simulink model "RadarSimulation"  (R2024a)
settings: Solver=VariableStepAuto  StartTime=0.0  StopTime=10.0  RelTol=1e-3
undefined symbols (not defined in the file or in its folder): physconst, pulseCoefficients
libraries: phasedenvlib x2, phasedtxrxlib x2, phaseddetectlib x1, dspxfrm3 x1
settings Model: Creator=Jayashre  LastModifiedBy=Jayashre

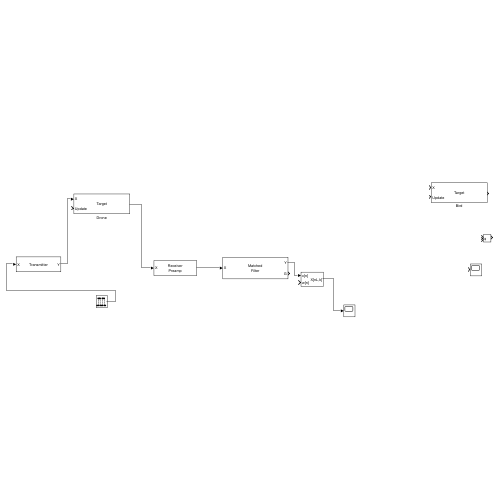
[thumbnail: Simulink's stored preview of the top-level diagram]
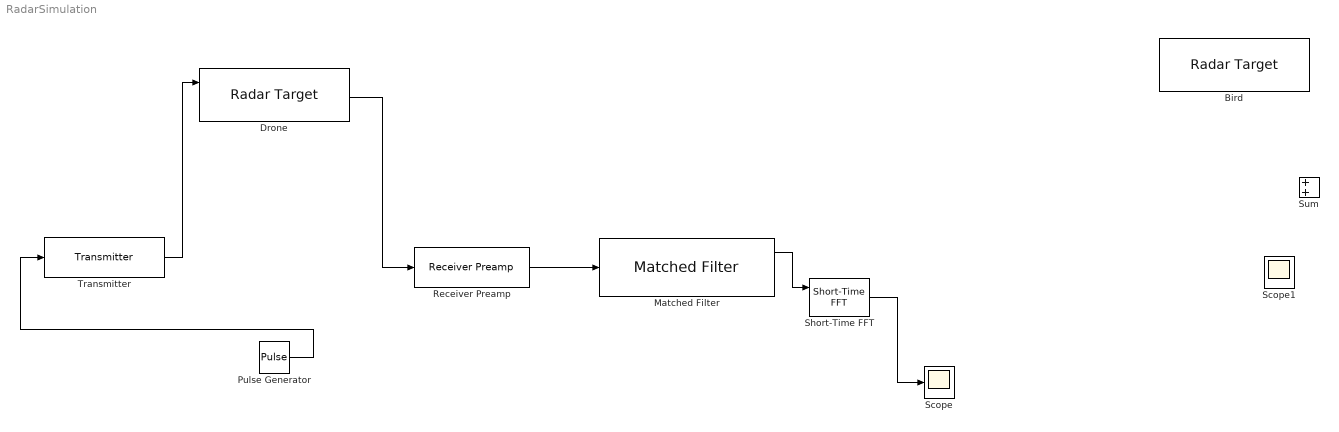
== system RadarSimulation ==
  Bird : phasedenvlib/Radar Target  EnablePolarization=off  Mode=Monostatic  MeanRCSSource=Property  ScatteringMatrixSource=Property  MeanRCS=0.01  ScatteringMatrix=eye( 2 )  Model=Swerling3  PropagationSpeed=physconst( 'LightSpeed' )  OperatingFrequency=1e10  SeedSource=Auto  Seed=0  SimulateUsing=Interpreted execution
  Drone : phasedenvlib/Radar Target  EnablePolarization=off  Mode=Monostatic  MeanRCSSource=Property  ScatteringMatrixSource=Property  MeanRCS=0.5  ScatteringMatrix=eye( 2 )  Model=Swerling2  PropagationSpeed=physconst( 'LightSpeed' )  OperatingFrequency=1e10  SeedSource=Auto  Seed=0  SimulateUsing=Interpreted execution
  Matched Filter : phaseddetectlib/Matched Filter  CoefficientsSource=Property  Coefficients=pulseCoefficients  SpectrumWindow=None  CustomSpectrumWindow=@hamming  SpectrumRange=[ 0, 1e5 ]  SampleRateFromInputCheckbox=on  SampleRate=1e6  SidelobeAttenuation=30  Beta=0.5  Nbar=4  GainOutputPort=on  MaximumNumInputSamplesSource=Auto  MaximumNumInputSamples=100  SimulateUsing=Interpreted execution
  Pulse Generator : DiscretePulseGenerator  Period=1000  PulseWidth=50  SampleTime=0.0001
  Receiver Preamp : phasedtxrxlib/Receiver Preamp  Gain=20  LossFactor=0  NoiseMethod=Noise temperature  NoiseFigure=0  ReferenceTemperature=290  SampleRateFromInputCheckbox=off  SampleRate=10000  NoisePower=0  EnableInputPort=off  PhaseNoiseInputPort=off  SeedSource=Auto  Seed=0  SimulateUsing=Interpreted execution
  Scope : Scope
  Scope1 : Scope
  Short-Time FFT : dspxfrm3/Short-Time FFT  W=256  OvLap=200  M=512
  Sum : Sum  Inputs=|++
  Transmitter : phasedtxrxlib/Transmitter  PeakPower=5000  GainMethod=Linear  Gain=20  LossFactor=0  OIP3=Inf  Table=[ -25, 5, -1; -10, 20, -2; 0, 27, 12; 5, 28, 12 ]  InUseOutputPort=off  CoherentOnTransmit=on  PhaseNoiseOutputPort=off  SimulateUsing=Interpreted execution  NoiseMethod=None  NoiseFigure=3  NoiseFactor=2  NoiseTemperature=290  ReferenceTemperature=290  SampleRate=1e6  SampleRateFromInputCheckbox=on  PhaseOffset=0  SeedSource=Auto  Seed=0
  wires:
  Receiver Preamp/1 -> Matched Filter/1
  Matched Filter/1 -> Short-Time FFT/1
  Short-Time FFT/1 -> Scope/1
  Drone/1 -> Receiver Preamp/1
  Pulse Generator/1 -> Transmitter/1
  Transmitter/1 -> Drone/1
